simulink model "flightControlSystem"  (R2024a)
settings: Solver=ode3  StartTime=0  StopTime=TFinal  FixedStep=Ts  RelTol=1e-3  EnableMultiTasking=on
undefined symbols (not defined in the file): codertarget, Controller, DiscIntNeverNeededParam, Discrete, Estimator, g, gray, init, orient_ref, pos_ref, Sensors, Time, Ts, var_acc_angle_N, var_bias_gyr_N, var_gyro_p_N, Vehicle
libraries: simulink x46, visiontextngfix x12, matrix_library x9, slpidlib x4, ctrlSharedLib x4, sharedtransform x3, visionconversions x1, parrotlib x1
(part 3 of 3)

== system flightControlSystem/Control System/State Estimator/XY Position Estimator/EstimatorVelocity/xy velocity w//o angular velocity compensation ==
  note: Optical flow raw readings are converted to velocity in m/s based on the estimated altitude
  optical_flow : Inport
  z_estimate : Inport  Port=2
  " " : Product  Inputs=**
  Compare To Constant : simulink/Logic and Bit Operations/Compare To Constant  relop=<  const=200*4  OutDataTypeStr=boolean
  Counter Free-Running : simulink/Sources/Counter Free-Running  NumBits=32  tsamp=-1
  Gain : Gain  Gain=-1
  Select dxy : Selector  InputPortWidth=3  IndexOptions=Index vector (dialog)  Indices=[1 2]  OutputSizes=1
  Switch : Switch  Criteria=u2 > Threshold  SaturateOnIntegerOverflow=off  InputSameDT=off
  opticalFlowErrorCorrect : Gain  Gain=1.15
  optical_flow_dx_dy : Outport
  wires:
  Select dxy/1 -> optical_flow_dx_dy/1  "optical_flow_dx_dy"
  " "/1 -> opticalFlowErrorCorrect/1
  opticalFlowErrorCorrect/1 -> Switch/3
  Gain/1 -> " "/2
  Switch/1 -> Select dxy/1
  Counter Free-Running/1 -> Compare To Constant/1
  Compare To Constant/1 -> Switch/2
  optical_flow/1 -> " "/1, Switch/1
  z_estimate/1 -> Gain/1

== matlab function flightControlSystem/Image Processing System/MATLAB Function1 ==
  data: imgin input; bw output; N output; ln1 output size=[10000 10000]; ln2 output size=[10000 10000]
function [bw , N, ln1, ln2] = imgprocessing(imgin)

greyimg=rgb2gray((imgin));
bw =( imbinarize(greyimg));
bw = bwareaopen(bw,30); %Remove niose less than 30 pixels
% se = strel('disk',2); % Fill a gap
% bw = imclose(uint32(bw),se); % Fill a gap
bw = imfill(bw,'holes'); % Fill any holes

% bw=imdilate(bwareaopen(bw,30),strel('disk', 20));


edg = edge(greyimg,'sobel');
edg = imdilate(edg,strel('disk',2));



[boundary ,~,N,~] = bwboundaries(edg);
perimeter=[];
for k=1:length(boundary)
  bound = boundary{k};
  delta_sq = diff(bound).^2;    
  perimeter = [perimeter; sum(sqrt(sum(delta_sq,2)))];
end

[~,n]=sort(perimeter ,'descend');
if N>=2
    ll1=boundary{n(1)};
    ll2=boundary{n(2)};
    ln1=[];
    for i=1:size(ll1,1)
        ln1=[ln1 ll1(i,2) ll1(i,1)];
    end
    ln2=[];
    for i=1:size(ll2,1)
        ln2=[ln2 ll2(i,2) ll2(i,1)];
    end
elseif isempty(n)~=1
    ll1=boundary{n(1)};
    ln1=[];
    for i=1:size(ll1,1)
        ln1=[ln1 ll1(i,2) ll1(i,1)];
    end
    ln2=ln1;
else
    ln1=[1 0 0 0 0 1 ];
    ln2=[1 0 0 0 0 1 ];
end

% disp(boundary)
% disp(perimeter)
% disp(ln1)
% disp(ln2)
% disp(n)

== matlab function flightControlSystem/Image Processing System/MATLAB Function2 ==
  data: bw input; roi_l input; roi_r input; center output size=[1 2]; roi output; blkroi output; area_l output; area_r output; centroid output; centroid_blk output; land output; blk_l input; blk_r input
function [center, roi, blkroi, area_l ,area_r, centroid, centroid_blk , land]= fcn(bw, roi_l, roi_r, blk_l, blk_r)

bw_l=roi_l.*bw;
bw_r=roi_r.*bw;
area_l=sum(sum(bw_l));
area_r=sum(sum(bw_r));
roi=bw_l+bw_r;
blk=blk_l.*blk_r;
blkroi=blk.*bw;


centroids= regionprops(roi, 'Centroid');

if isempty(centroids)==1
    centroid=[81 60];
elseif isstruct(centroids)==1
    centroid=centroids(1).Centroid;
else
    centroid=centroids;
end

centroids= regionprops(blkroi, 'Centroid');

if isempty(centroids)==1
    centroid_blk=[81 60];
elseif isstruct(centroids)==1
    centroid_blk=centroids(1).Centroid;
else
    centroid_blk=centroids;
end

[centers] = ( imfindcircles(bw,[15 25], 'ObjectPolarity','bright'));
centers1=imfindcircles(bw,[25 35], 'ObjectPolarity','bright');
centers2=imfindcircles(bw,[35 45], 'ObjectPolarity','bright');
centers3=imfindcircles(bw,[45 55], 'ObjectPolarity','bright');
centers4=imfindcircles(bw,[55 70], 'ObjectPolarity','bright');
if isempty(centers)==1
    if isempty(centers1)==1
        if isempty(centers2)==1
            if isempty(centers3)==1
                if isempty(centers4)==1
                    center=[200,200];
                else
                    center=[centers4(1) centers4(2)];
                end
            else
                 center=[centers3(1) centers3(2)];
            end 
        else
             center=[centers2(1) centers2(2)];
        end 
    else
         center=[centers1(1) centers1(2)];
    end 
else
    center=[centers(1) centers(2)];
end


landmark=zeros(120,160);
if center(1)~=200
    landmark(uint8(center(2)),uint8(center(1)))=1;
end

land=sum(sum(landmark.*roi_l))+sum(sum(landmark.*roi_r));
if land>0
    land=1;
end

== matlab function flightControlSystem/Image Processing System/MATLAB Function3 ==
  data: pathold input; N input; centroid input; centroid_blk input; area_l input; area_r input; roiangle output; angle input; roicord_l output size=[1 6]; roicord_r output size=[1 6]; blackcord_l output; blackcord_r output; speed output
function [roiangle, roicord_l, roicord_r,blackcord_l , blackcord_r, speed] = roi( pathold, N, centroid, centroid_blk, area_l, area_r, angle)
path=[centroid 80 60];
% [row,~]=size(path);
x=[80 60];
y=[path(1,1) path(1,2)];
d1=norm(x-y);
y=[path(1,3) path(1,4)];
d2=norm(x-y);
x=[path(1,1) path(1,2)];
y=[80 60];
pathdis=norm(x-y)
if pathdis<6 && pathdis >=4
    speed=0.2;
elseif pathdis<4
    path=[centroid_blk 80 60];
    speed=0.5;
elseif pathdis<20 && pathdis >=10
    speed=pathdis/500
else
    speed=pathdis/250
end

if (pathold(1,1)+pathold(1,2)+pathold(1,3)+pathold(1,4))~=0
pendis=abs((pathold(1,3) - pathold(1,1)) * (pathold(1,2) - 60) - (pathold(1,1) - 80) * (pathold(1,4) - pathold(1,2)))./sqrt((pathold(1,3) - pathold(1,1)) ^ 2 + (pathold(1,4) - pathold(1,2)) ^ 2)
x=[pathold(1,1) pathold(1,3)];
y=[pathold(1,2) pathold(1,4)];
pathdisold=norm(x-y);
anglecorr=pendis/pathdisold;
pendis_cen=abs((pathold(1,3) - pathold(1,1)) * (pathold(1,2) - centroid(2)) - (pathold(1,1) - centroid(1)) * (pathold(1,4) - pathold(1,2)))./sqrt((pathold(1,3) - pathold(1,1)) ^ 2 + (pathold(1,4) - pathold(1,2)) ^ 2)
    if (pendis<= 10 || (pendis>= 10 && pendis_cen>=5)) && pathdis ~=1
    
    
    if   (path(1,1)+path(1,2)+path(1,3)+path(1,4))~=0 && d1>=d2 
    
    %     x0=path(2,1);
    %     y0=path(2,2);
    %     x1=path(2,3);
    %     y1=path(2,4);
    %     x2=path(2,1);
    %     y2=30;
    %     x10 = x1-x0;
    %     y10 = y1-y0;
    %     x20 = x2-x0;
    %     y20 = y2-y0; 
    %     roiangle = (atan2(abs(x10*y20-x20*y10),x10*y10+x20*y20));
    
        pendis=abs((path(1,3) - path(1,1)) * (path(1,2) - 60) - (path(1,1) - 80) * (path(1,4) - path(1,2)))./sqrt((path(1,3) - path(1,1)) ^ 2 + (path(1,4) - path(1,2)) ^ 2);
        x=[path(1,1) path(1,3)];
        y=[path(1,2) path(1,4)];
        pathdis=norm(x-y);
        anglecorr=pendis/pathdis;
    
        a = [-80*(path(1,3)-path(1,1)) - 60*(path(1,4)-path(1,2)) ;  -path(1,2)*(path(1,3)-path(1,1)) + path(1,1)*(path(1,4)-path(1,2))]; 
        b = [path(1,3) - path(1,1), path(1,4) - path(1,2) ;  path(1,2) - path(1,4), path(1,3) - path(1,1)];
        projpoint = -(b\a)-[80,60];
    
        if projpoint(1)<0 && angle>-1.5708 && angle<1.5708
            anglecorr=-anglecorr;
        elseif  projpoint(1)>0 && (angle<-1.5708 || angle>1.5708)
            anglecorr=-anglecorr;
        elseif projpoint(1)==0 && projpoint(2)>0 && angle==1.5708 
            anglecorr=-anglecorr;
        elseif projpoint(1)==0 && projpoint(2)<0 && angle==-1.5708 
            anglecorr=-anglecorr;
        end
    
    
        v1 = [path(1,3) - path(1,1) , path( 1,4)- path(1,2)];
        v2 = [ 0, 1];
        roiangle = acos(dot(v1,v2)/(norm(v1)*norm(v2))) +anglecorr;
        
        if path(1,1)<80
            roiangle=-roiangle;
        end
    
        
    elseif  (path(1,1)+path(1,2)+path(1,3)+path(1,4))~=0 && d2>=d1 
    
        pendis=abs((path(1,3) - path(1,1)) * (path(1,2) - 60) - (path(1,1) - 80) * (path(1,4) - path(1,2)))./sqrt((path(1,3) - path(1,1)) ^ 2 + (path(1,4) - path(1,2)) ^ 2);
        x=[path(1,1) path(1,3)];
        y=[path(1,2) path(1,4)];
        pathdis=norm(x-y);
        anglecorr=pendis/pathdis;
    
        a = [-80*(path(1,3)-path(1,1)) - 60*(path(1,4)-path(1,2)) ;  -path(1,2)*(path(1,3)-path(1,1)) + path(1,1)*(path(1,4)-path(1,2))]; 
        b = [path(1,3) - path(1,1), path(1,4) - path(1,2) ;  path(1,2) - path(1,4), path(1,3) - path(1,1)];
        projpoint = -(b\a)-[80,60];
    
        if projpoint(1)<0 && angle>-1.5708 && angle<1.5708
            anglecorr=-anglecorr;
        elseif  projpoint(1)>0 && (angle<-1.5708 || angle>1.5708)
            anglecorr=-anglecorr;
        elseif projpoint(1)==0 && projpoint(2)>0 && angle==1.5708 
            anglecorr=-anglecorr;
        elseif projpoint(1)==0 && projpoint(2)<0 && angle==-1.5708 
            anglecorr=-anglecorr;
        end
    
        v1 = [path(1,1) - path(1,3) , path( 1,2)- path(1,4)];
        v2 = [ 0, 1];
        roiangle = acos(dot(v1,v2)/(norm(v1)*norm(v2))) +anglecorr;
    
        if path(1,1)<80
            roiangle=-roiangle;
        end
    
    
    
    elseif (path(1,1)+path(1,2)+path(1,3)+path(1,4))~=0
    
        pendis=abs((path(1,3) - path(1,1)) * (path(1,2) - 60) - (path(1,1) - 80) * (path(1,4) - path(1,2)))./sqrt((path(1,3) - path(1,1)) ^ 2 + (path(1,4) - path(1,2)) ^ 2);
        x=[path(1,1) path(1,3)];
        y=[path(1,2) path(1,4)];
        pathdis=norm(x-y);
        anglecorr=pendis/pathdis;
    
        a = [-80*(path(1,3)-path(1,1)) - 60*(path(1,4)-path(1,2)) ;  -path(1,2)*(path(1,3)-path(1,1)) + path(1,1)*(path(1,4)-path(1,2))]; 
        b = [path(1,3) - path(1,1), path(1,4) - path(1,2) ;  path(1,2) - path(1,4), path(1,3) - path(1,1)];
        projpoint = -(b\a)-[80,60];
    
        if projpoint(1)<0 && angle>-1.5708 && angle<1.5708
            anglecorr=-anglecorr;
        elseif  projpoint(1)>0 && (angle<-1.5708 || angle>1.5708)
            anglecorr=-anglecorr;
        elseif projpoint(1)==0 && projpoint(2)>0 && angle==1.5708 
            anglecorr=-anglecorr;
        elseif projpoint(1)==0 && projpoint(2)<0 && angle==-1.5708 
            anglecorr=-anglecorr;
        end
    
        v1 = [path(1,3) - path(1,1) , path( 1,4)- path(1,2)];
        v2 = [ 0, path(1,1) - path(1,2)];
        roiangle = acos(dot(v1,v2)/(norm(v1)*norm(v2))) +anglecorr;
    
    
    else
    
    %     angle=angle*180/(1*pi);
    %     diff=abs(area_l-area_r)/10;
    %     if area_l>area_r
    %         angle=angle-1*diff;
    %     else
    %         angle=angle+1*diff;
    %     end 
    %     if area_r+area_l==0
    %         speed=-0.2;
    %     elseif area_r+area_l<750 && area_r+area_l>550
    %         speed=0.2;
    %     else
    %         speed=0.3;
    %     end
    %     roiangle=angle*pi/180;
    
    %     if path~=[0 0 0 0]
    %         x0=path(1,1);
    %         y0=path(1,2);
    %         x1=path(1,3);
    %         y1=path(1,4);
    %         x2=path(1,1);
    %         y2=30;
    %         x10 = x1-x0;
    %         y10 = y1-y0;
    %         x20 = x2-x0;
    %         y20 = y2-y0; 
    %         roiangle = (atan2(abs(x10*y20-x20*y10),x10*y10+x20*y20));
    
            % v1 = [x1 - x2, y1 - y2]
            % v2 = [x3 - x2, Y3 - y2]
    %         v1 = [path(1,3) - path(1,1) , path( 1,4)- path(1,2)];
    %         v2 = [ 0, path(1,1) - path(1,2)];
    %         roiangle = acos(dot(v1,v2)/(norm(v1)*norm(v2)));
    
    %     else
            roiangle=angle;
    %     end
        speed=0.3;
    end
    
    
    
    % disp(roiangle)
    % disp(anglecorr)
    
    
    % 
    % if abs(area_l-area_r)<200
    % 
    % 
    %     x=[path(1,1) path(1,3)];
    %     y=[path(1,2) path(1,4)];
    %     speed=norm(x-y)/300;
    % 
    % 
    %     pendis=abs((path(1,3) - path(1,1)) * (path(1,2) - 60) - (path(1,1) - 80) * (path(1,4) - path(1,2)))./sqrt((path(1,3) - path(1,1)) ^ 2 + (path(1,4) - path(1,2)) ^ 2);
    %     x=[path(1,1) path(1,3)];
    %     y=[path(1,2) path(1,4)];
    %     pathdis=norm(x-y);
    %     anglecorr=pendis/pathdis;
    % 
    %     a = [-80*(path(1,3)-path(1,1)) - 60*(path(1,4)-path(1,2)) ;  -path(1,2)*(path(1,3)-path(1,1)) + path(1,1)*(path(1,4)-path(1,2))]; 
    %     b = [path(1,3) - path(1,1), path(1,4) - path(1,2) ;  path(1,2) - path(1,4), path(1,3) - path(1,1)];
    %     projpoint = -(b\a)-[80,60];
    % 
    %     if projpoint(1)<0 && angle>-1.5708 && angle<1.5708
    %         anglecorr=-anglecorr;
    %     elseif  projpoint(1)>0 && (angle<-1.5708 || angle>1.5708)
    %         anglecorr=-anglecorr;
    %     elseif projpoint(1)==0 && projpoint(2)>0 && angle==1.5708 
    %         anglecorr=-anglecorr;
    %     elseif projpoint(1)==0 && projpoint(2)<0 && angle==-1.5708 
    %         anglecorr=-anglecorr;
    %     end


    else
        a = [-80*(pathold(1,3)-pathold(1,1)) - 60*(pathold(1,4)-pathold(1,2)) ;  -pathold(1,2)*(pathold(1,3)-pathold(1,1)) + pathold(1,1)*(pathold(1,4)-pathold(1,2))]; 
        b = [pathold(1,3) - pathold(1,1), pathold(1,4) - pathold(1,2) ;  pathold(1,2) - pathold(1,4), pathold(1,3) - pathold(1,1)];
        projpoint = -(b\a)-[80,60];
    
        if projpoint(1)<0 && angle>-1.5708 && angle<1.5708
            anglecorr=-anglecorr;
        elseif  projpoint(1)>0 && (angle<-1.5708 || angle>1.5708)
            anglecorr=-anglecorr;
        elseif projpoint(1)==0 && projpoint(2)>0 && angle==1.5708 
            anglecorr=-anglecorr;
        elseif projpoint(1)==0 && projpoint(2)<0 && angle==-1.5708 
            anglecorr=-anglecorr;
        end
    
        roiangle=angle+anglecorr/10;
        speed=0.3;
    end
else
    roiangle=angle;
    speed=0.2;
end






n=10;
m=25;
l=25;
xc=80;
yc=60;

x0=xc-l*sin(roiangle);
y0=yc+l*cos(roiangle);
x1=xc+m*sin(roiangle);
y1=yc-m*cos(roiangle);
xr=x1+n*(y0-y1)/m;
yr=y1+n*(x1-x0)/m;
xl=x1-n*(y0-y1)/m;
yl=y1-n*(x1-x0)/m;


roicord_l=[x0 y0 xl yl x1 y1] ;
roicord_r=[x0 y0 x1 y1 xr yr];


n=60;
m=100;
l=0;
xc=80;
yc=60;


x0=xc-l*sin(roiangle+pi);
y0=yc+l*cos(roiangle+pi);
x1=xc+m*sin(roiangle+pi);
y1=yc-m*cos(roiangle+pi);
xr=x1+n*(y0-y1)/m;
yr=y1+n*(x1-x0)/m;
xl=x1-n*(y0-y1)/m;
yl=y1-n*(x1-x0)/m;


blackcord_l=[x0 y0 xl yl x1 y1] ;
blackcord_r=[x0 y0 x1 y1 xr yr];

== matlab function flightControlSystem/Image Processing System/MATLAB Function4 ==
  data: ln1 input; line output size=[100 100]; ln2 input; path output size=[100 100]
function [ line, path] = detectline(ln1, ln2)

[H,T,R] = hough(ln1);
P  = houghpeaks(H,5,'threshold',ceil(0.3*max(H(:))));
lines1 = houghlines(ln1,T,R,P,'FillGap',30,'MinLength',30);

if isempty(lines1)~=1
    line1=[];
    [~,col ]=size(lines1);
    linestart=[lines1.point1];
    lineend=[lines1.point2];
    for i = 1:1:col
        line1=[line1 ;[linestart(2*i-1) linestart(2*i) lineend(2*i-1) lineend(2*i) ]];        
    end
else
    line1=[0 0 0 0 ];
end


[H,T,R] = hough(ln2);
P  = houghpeaks(H,5,'threshold',ceil(0.3*max(H(:))));
lines2 = houghlines(ln2,T,R,P,'FillGap',30,'MinLength',30);


if isempty(lines2)~=1
    line2=[];
    [~,col ]=size(lines2);
    linestart=[lines2.point1];
    lineend=[lines2.point2];
    for i = 1:1:col
        line2=[line2 ;[linestart(2*i-1) linestart(2*i) lineend(2*i-1) lineend(2*i) ]];        
    end
else
    line2=[0 0 0 0 ];
end

path1=( line1(1,1)+line2(1,1))/2 ;
path2=( line1(1,2)+line2(1,2))/2 ;
path3=( line1(1,3)+line2(1,3))/2 ;
path4=( line1(1,4)+line2(1,4))/2 ;
path = [ path1 path2 path3 path4 ];

line=[line1 ; line2];
% angle=lines1.theta;
% disp(line)
% disp (path)

== stateflow chart flightControlSystem/Control System/Path Planning/Chart1 ==
  state Following_The_Line [group]
    state RotationForM_2
      entry:
      rot=true;
      during:
      xout = xout;
      yout=yout;
    state MoveForward
      entry:
      rot=false;
      during:
      dx=vel*cos(yawin);
      dy=vel*sin(yawin);
      xout=xout+dx;
      yout=yout+dy;
    state RotationOrLand
      entry:
      rot=false;
      during:
      xout = xout;
      yout=yout;
      zout=zout;
    state Turning
      entry:
      rot=false;
      during:
      xout=xout;
      yout=yout;
      zout=zout;
    RotationOrLand -> RotationForM_2 [order 1] : [L==true||R==true||LS==true||RS==true||L1==true||R1==true&&C==true]
    MoveForward -> Turning [order 1] : [M==false]
    Turning -> RotationOrLand [order 2] : [after(0.6,sec)&&C==true]
  state Starting_The_Drone [group]
    state RotationForM_1
      entry:
      rot=true;
      during:
      xout = xout;
      yout=yout;
      zout=zout;
    state Hover
      entry:
      land_1=0;
      rot=false;
      during:
      xout=0;
      yout=0;
      zout = -1.1;
    state LineFound
      entry:
      dx=0;
      dy=0;
      during:
      dx=vel*cos(yawin);
      dy=vel*sin(yawin);
      xout=xout+dx;
      yout=yout+dy;
    state RotationForM
      entry:
      rot=true;
      during:
      xout = xout;
      yout=yout;
    state FindLine
      during:
      dx=vel*cos(yawin);
      dy=vel*sin(yawin);
      xout=xout+dx;
      yout=yout+dy;
    (default) -> Hover
    RotationForM_1 -> RotationForM [order 2] : [C==false]{rot==false}
    FindLine -> RotationForM_1 : [C==true]
    Hover -> LineFound : [after(2,sec)]{rot=true}
    LineFound -> RotationForM [order 2] : [O==true]
    RotationForM -> FindLine [order 1] : [M==true]{rot==false}
  state Landing_The_Drone [group]
    state Land
      entry:
      land_1=1;
  RotationForM_1 -> Land [order 3] : [land==1]
  RotationForM_2 -> RotationForM_1 [order 3] : [M==true&&C==true]
  RotationForM_1 -> MoveForward [order 1] : [M==true&&C==true]{rot==false}
  RotationForM_2 -> Land [order 1] : [land==1]
  RotationForM_2 -> FindLine [order 2] : [C==false]
  LineFound -> MoveForward [order 1] : [M==true&&C==true]
  MoveForward -> FindLine [order 2] : [C==false]
  RotationForM -> Land [order 2] : [land==1]
  RotationOrLand -> Land [order 2] : [land==1]
  RotationOrLand -> FindLine [order 3] : [C==false]
  Turning -> FindLine [order 1] : [C==false]
  data: L input; M input; R input; LS input; C input; RS input; L1 input; R1 input; O input; land input; center input; xout output; yout output; zout output; rot output; yawin input; dy local; dx local; vel constant double =4.5*10^-4; land_1 output

== stateflow chart flightControlSystem/Control System/Path Planning/Chart2 ==
  state STEER
    entry:
    OUT=0;
    during:
    if(L==true)
    OUT=-1;
    elseif(R==true)
    OUT=1;
    elseif(L1==true)
    OUT=-1;
    elseif(R1==true)
    OUT=1;
    elseif(LS==true)
    OUT=-1;
    elseif(RS==true)
    OUT=1;
    else
    OUT=0;
    end
  (default) -> STEER
  data: L input; R input; L1 input; R1 input; LS input; RS input; OUT output

== matlab function flightControlSystem/Control System/Path Planning/MATLAB Function ==
  data: x output; aX_ input; y output; aY_ input; aZ_ input; cx input; cy input; z output
function [x,y,z] = land(aX_, aY_,  aZ_, cx, cy)
if cx<=85 && cx>=75 && cy<=65 && cy>=55
    x=aX_;
    y=aY_;
    z=aZ_+0.1;
elseif cx>=85 && cx~=200 
    y=aY_+0.08;
    z=aZ_;
    if cy>=75 && cy~=200
        x=aX_-0.06;
    elseif  cy<=55 && cy~=200  
        x=aX_+0.06;
    else
        x=aX_;
    end 
elseif cx<=75&&cx~=200
    y=aY_-0.08;
    z=aZ_;
    if cy>=65 && cy~=200
        x=aX_-0.06;
    elseif  cy<=55 && cy~=200  
        x=aX_+0.06;
    else
        x=aX_;
    end 
else
    x=aX_;
    y=aY_;
    z=aZ_+0.2;
end 

% flag=flag1;
% if data==0 && flag==0
%     land=1;
%     flag=0;
% else
%     land=0;
% end

== matlab function flightControlSystem/Control System/Controller/Position Controller/Position error transformation (Earth to Body frame) ==
  data: yaw input; xy_err_earth input; xy_err_body output
function xy_err_body = fcn(yaw,xy_err_earth)

transformation = [cos(yaw), sin(yaw); -sin(yaw),  cos(yaw)];
xy_err_body = transformation * xy_err_earth;


end

== matlab function flightControlSystem/Image Processing System/MATLAB Function ==
  data: RGB input; masked output
function masked  = createMask(RGB)
%createMask  Threshold RGB image using auto-generated code from colorThresholder app.
%  [BW,MASKEDRGBIMAGE] = createMask(RGB) thresholds image RGB using
%  auto-generated code from the colorThresholder app. The colorspace and
%  range for each channel of the colorspace were set within the app. The
%  segmentation mask is returned in BW, and a composite of the mask and
%  original RGB images is returned in maskedRGBImage.

% Auto-generated by colorThresholder app on 31-Jul-2022
%------------------------------------------------------


% Convert RGB image to chosen color space
I = RGB;

% Define thresholds for channel 1 based on histogram settings
channel1Min = 125.000;
channel1Max = 255.000;

% Define thresholds for channel 2 based on histogram settings
channel2Min = 0.000;
channel2Max = 119.000;

% Define thresholds for channel 3 based on histogram settings
channel3Min = 0.000;
channel3Max = 116.000;

% Create mask based on chosen histogram thresholds
sliderBW = (I(:,:,1) >= channel1Min ) & (I(:,:,1) <= channel1Max) & ...
    (I(:,:,2) >= channel2Min ) & (I(:,:,2) <= channel2Max) & ...
    (I(:,:,3) >= channel3Min ) & (I(:,:,3) <= channel3Max);
BW = sliderBW;

% Initialize output masked image based on input image.
masked = RGB;

% Set background pixels where BW is false to zero.
masked(repmat(~BW,[1 1 3])) = 0;

end
